simulink model "Switch_Led_Sys"  (R2018b)
settings: Solver=VariableStepAuto  StartTime=0.0  StopTime=inf  RelTol=1e-3
libraries: simulink x1
settings Model: Creator=lenovo2  LastModifiedBy=lenovo2

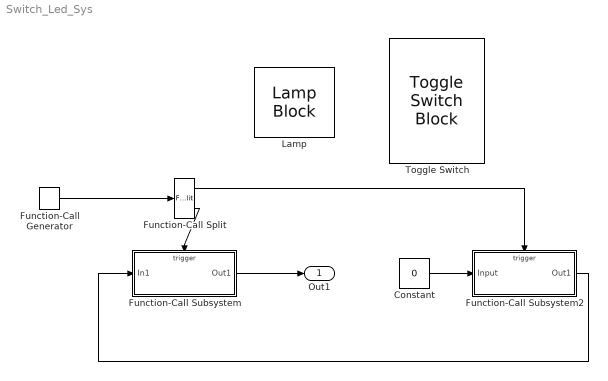
== system Switch_Led_Sys ==
  Constant : Constant  Value=0
  Function-Call Generator : simulink/Ports & Subsystems/Function-Call Generator  sample_time=1  numberOfIterations=1
  Function-Call Split : FunctionCallSplit  NumOutputPorts=2  OutputPortLayout=default
  Function-Call Subsystem : Subsystem  TreatAsAtomicUnit=on
  Function-Call Subsystem2 : Subsystem  TreatAsAtomicUnit=on
  Lamp : LampBlock  WebBlockId=31
  Toggle Switch : ToggleSwitchBlock  WebBlockId=30
      settings: Values={{'Off', 'On'}, [0 1]}
  Out1 : Outport
  wires:
  Function-Call Generator/1 -> Function-Call Split/1
  Function-Call Subsystem/1(Out1) -> Out1/1
  Function-Call Split/1 -> Function-Call Subsystem2/Trigger
  Function-Call Subsystem2/1(Out1) -> Function-Call Subsystem/1(In1)
  Function-Call Split/2 -> Function-Call Subsystem/Trigger
  Constant/1 -> Function-Call Subsystem2/1(Input)

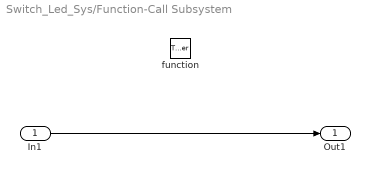
== system Switch_Led_Sys/Function-Call Subsystem ==
  In1 : Inport
  function : TriggerPort  TriggerType=function-call  VariantControl=Variant
  Out1 : Outport
  wires:
  In1/1 -> Out1/1

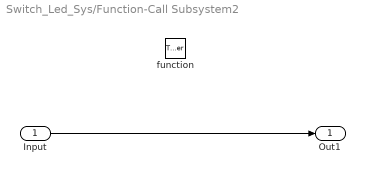
== system Switch_Led_Sys/Function-Call Subsystem2 ==
  Input : Inport
  function : TriggerPort  TriggerType=function-call  VariantControl=Variant
  Out1 : Outport
  wires:
  Input/1 -> Out1/1
